simulink subsystem "inv_clarke"  (R2022b)
settings: Solver=VariableStepAuto  StartTime=0.0  StopTime=10.0  RelTol=1e-3
settings Model: Creator=jack  LastModifiedBy=jack

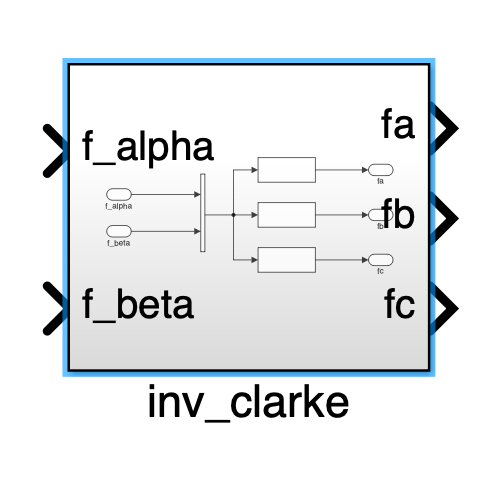
[thumbnail: Simulink's stored preview of the top-level diagram]
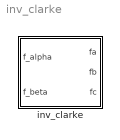
== system inv_clarke ==
  inv_clarke : Subsystem

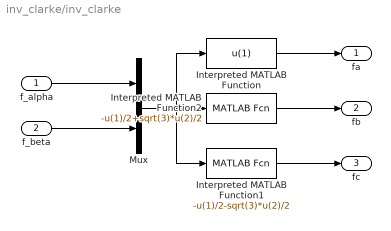
== system inv_clarke/inv_clarke ==
  f_alpha : Inport
  f_beta : Inport  Port=2
  Interpreted MATLAB Function : MATLABFcn  MATLABFcn=u(1)
  Interpreted MATLAB Function1 : MATLABFcn  MATLABFcn=-u(1)/2-sqrt(3)*u(2)/2
  Interpreted MATLAB Function2 : MATLABFcn  MATLABFcn=-u(1)/2+sqrt(3)*u(2)/2
  Mux : Mux  Inputs=2
  fa : Outport
  fb : Outport  Port=2
  fc : Outport  Port=3
  wires:
  Mux/1 -> Interpreted MATLAB Function/1, Interpreted MATLAB Function2/1, Interpreted MATLAB Function1/1
  f_alpha/1 -> Mux/1
  f_beta/1 -> Mux/2
  Interpreted MATLAB Function/1 -> fa/1
  Interpreted MATLAB Function2/1 -> fb/1
  Interpreted MATLAB Function1/1 -> fc/1
